simulink model "Ensamblaje2"  (R2018b)
settings: Solver=VariableStepAuto  StartTime=0.0  StopTime=30  RelTol=1e-6
model workspace: external: MATLAB File C:\matlabbb\EnsamblajePrueba_DataFile.m (data not in the file)
values from neighbouring files (symbols this model uses):
  m = [5.70044 3.22698 4.31272 2.07206 2.24665 1.60879]    [Modelo.m]    (also in robot_init.m; robotics_toolbox.m)
undefined symbols (not defined in the file or in its folder): smiData, X, Y, Z
libraries: sm_lib x40, nesl_utility x15, simulink x1
settings Model: Creator=aland  LastModifiedBy=aland

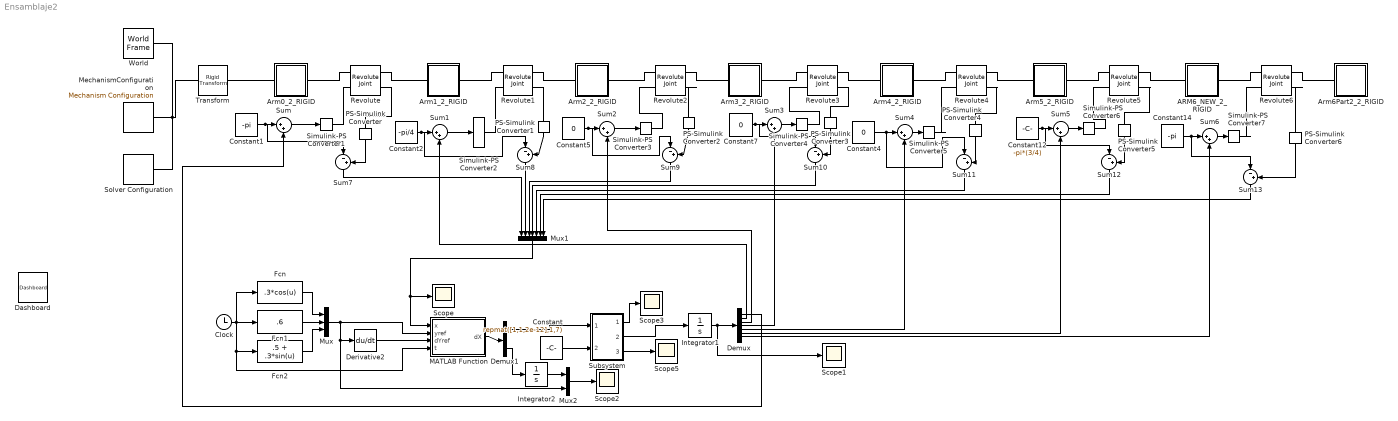
== system Ensamblaje2 ==
  ARM6_NEW_2_RIGID : Subsystem
  Arm0_2_RIGID : Subsystem
  Arm1_2_RIGID : Subsystem
  Arm2_2_RIGID : Subsystem
  Arm3_2_RIGID : Subsystem
  Arm4_2_RIGID : Subsystem
  Arm5_2_RIGID : Subsystem
  Arm6Part2_2_RIGID : Subsystem
  Clock : Clock
      settings: Decimation=10000
  Constant : Constant  Value=repmat([1,1,2e-12],1,7)
  Constant1 : Constant  Value=-pi
  Constant12 : Constant  Value=-pi*(3/4)
  Constant14 : Constant  Value=-pi
  Constant2 : Constant  Value=-pi/4
  Constant4 : Constant  Value=0
  Constant5 : Constant  Value=0
  Constant7 : Constant  Value=0
  Dashboard : simulink/Dashboard  SystemSampleTime=-1
      settings: SourceProductName=Simulink  SourceProductBaseCode=SL
  Demux : Demux  Outputs=7
  Demux1 : Demux  Outputs=[7 3]
  Derivative2 : Derivative
  Fcn : Fcn  Expr=.3*cos(u)
  Fcn1 : Fcn  Expr=.6
  Fcn2 : Fcn  Expr=.5 + .3*sin(u)
  Integrator1 : Integrator  InitialCondition=[0 0 0 0 0 0 0]  UpperSaturationLimit=4  LowerSaturationLimit=-4
  Integrator2 : Integrator  InitialCondition=[.148 0 1.2385]  UpperSaturationLimit=4  LowerSaturationLimit=-4
  MATLAB Function : MATLAB Function  TreatAsAtomicUnit=on
  MechanismConfiguration : sm_lib/Utilities/Mechanism Configuration  UniformGravity=Constant  GravityVector=[0 -9.80665 0]  GravityUnits=m/s^2  LinearizationDelta=0.001
  Mux : Mux  Inputs=3
  Mux1 : Mux  Inputs=7
  Mux2 : Mux  Inputs=2
  PS-Simulink Converter{,1..6} (7 alike) : nesl_utility/PS-Simulink Converter  PhysicalDomain=network_engine_domain  SubClassName=ps_output  LeftPortType=input  RightPortType=output  PseudoPeriodic=off  Frequencies=[]  Unit=1  AffineConversion=off
  Revolute{,1..4} (5 alike) : sm_lib/Joints/Revolute Joint  SenseConstraintForce=off  SenseConstraintForceX=off  SenseConstraintForceY=off  SenseConstraintForceZ=off  SenseConstraintTorque=off  SenseConstraintTorqueX=off  SenseConstraintTorqueY=off  SenseConstraintTorqueZ=off  SenseTotalForce=off  SenseTotalForceX=off  SenseTotalForceY=off  SenseTotalForceZ=off  SenseTotalTorque=off  SenseTotalTorqueX=off  SenseTotalTorqueY=off  SenseTotalTorqueZ=off  CompositeWrenchDir=FollowerOnBase  CompositeWrenchFrame=BaseFrame  EquilibriumPosition=0  EquilibriumPositionUnits=rad  SpringStiffness=0  SpringStiffnessUnits=N*m/rad  DampingCoefficient=0  DampingCoefficientUnits=N*m/(rad/s)  TorqueActuationMode=ComputedTorque  MotionActuationMode=InputMotion  SensePosition=on  SenseVelocity=off  SenseAcceleration=off  SenseTorqueForce=off  PositionTargetSpecify=off  PositionTargetPriority=Low  PositionTargetValue=0  PositionTargetValueUnits=deg  VelocityTargetSpecify=off  VelocityTargetPriority=High  VelocityTargetValue=0  VelocityTargetValueUnits=deg/s
  Revolute5 : sm_lib/Joints/Revolute Joint  SenseConstraintForce=off  SenseConstraintForceX=off  SenseConstraintForceY=off  SenseConstraintForceZ=off  SenseConstraintTorque=off  SenseConstraintTorqueX=off  SenseConstraintTorqueY=off  SenseConstraintTorqueZ=off  SenseTotalForce=off  SenseTotalForceX=off  SenseTotalForceY=off  SenseTotalForceZ=off  SenseTotalTorque=off  SenseTotalTorqueX=off  SenseTotalTorqueY=off  SenseTotalTorqueZ=off  CompositeWrenchDir=FollowerOnBase  CompositeWrenchFrame=BaseFrame  EquilibriumPosition=0  EquilibriumPositionUnits=rad  SpringStiffness=0  SpringStiffnessUnits=N*m/rad  DampingCoefficient=0  DampingCoefficientUnits=N*m/(rad/s)  TorqueActuationMode=ComputedTorque  MotionActuationMode=InputMotion  SensePosition=on  SenseVelocity=off  SenseAcceleration=off  SenseTorqueForce=off  PositionTargetSpecify=off  PositionTargetPriority=Low  PositionTargetValue=smiData.RevoluteJoint(6).Rz.Pos  PositionTargetValueUnits=deg  VelocityTargetSpecify=off  VelocityTargetPriority=High  VelocityTargetValue=0  VelocityTargetValueUnits=deg/s
  Revolute6 : sm_lib/Joints/Revolute Joint  SenseConstraintForce=off  SenseConstraintForceX=off  SenseConstraintForceY=off  SenseConstraintForceZ=off  SenseConstraintTorque=off  SenseConstraintTorqueX=off  SenseConstraintTorqueY=off  SenseConstraintTorqueZ=off  SenseTotalForce=off  SenseTotalForceX=off  SenseTotalForceY=off  SenseTotalForceZ=off  SenseTotalTorque=off  SenseTotalTorqueX=off  SenseTotalTorqueY=off  SenseTotalTorqueZ=off  CompositeWrenchDir=FollowerOnBase  CompositeWrenchFrame=BaseFrame  EquilibriumPosition=0  EquilibriumPositionUnits=rad  SpringStiffness=0  SpringStiffnessUnits=N*m/rad  DampingCoefficient=0  DampingCoefficientUnits=N*m/(rad/s)  TorqueActuationMode=ComputedTorque  MotionActuationMode=InputMotion  SensePosition=on  SenseVelocity=off  SenseAcceleration=off  SenseTorqueForce=off  PositionTargetSpecify=off  PositionTargetPriority=Low  PositionTargetValue=smiData.RevoluteJoint(7).Rz.Pos  PositionTargetValueUnits=deg  VelocityTargetSpecify=off  VelocityTargetPriority=High  VelocityTargetValue=0  VelocityTargetValueUnits=deg/s
  Scope{,1..3,5} (5 alike) : Scope
  Simulink-PS Converter{1..7} (7 alike) : nesl_utility/Simulink-PS Converter  PhysicalDomain=network_engine_domain  SubClassName=ps_input  LeftPortType=input  RightPortType=output  PseudoPeriodic=off  Frequencies=[]  NoiseDistribution=none  NoiseParameters=[]  Unit=1  AffineConversion=off  FilteringAndDerivatives=filter  SimscapeFilterOrder=2  InputFilterTimeConstant=0.0001  UdotUserProvided=0
  Solver Configuration : nesl_utility/Solver Configuration  PhysicalDomain=network_engine_domain  SubClassName=solver  LeftPortType=input  RightPortType=generic  Tones=[]  Harmonics=[]  SimulateNoise=off  Profile=off  UseLocalSampling=off  EnableSwitchedLinearOptims=on  FrequencyDomain=off  UseCCode=off  RelTol=0.001  AbsTol=1e-06  MinStep=1e-09  ToWorkspace=off  RevertToSquareIcSolve=off  NumHomotopyIterations=100  PhasorMode=off  PhasorModeNumHarmonics=1  DoDC=off  ResidualTolerance=1e-09  UseLocalSolver=off  LocalSolverChoice=NE_BACKWARD_EULER_ADVANCER  LocalSolverSampleTime=0.001  DoFixedCost=off  MaxNonlinIter=3  MaxModeIter=2  LinearAlgebra=auto  EquationFormulation=NE_TIME_EF  DelaysMemoryBudget=1024  AutomaticFiltering=on  FilteringTimeConstant=0.001  PartitionStorageMethod=AS_NEEDED  PartitionMemoryBudget=1024
  Subsystem : Subsystem
  Sum{,1..6} (7 alike) : Sum  Inputs=|++
  Sum{7..13} (7 alike) : Sum  Inputs=|-+
  Transform : sm_lib/Frames and Transforms/Rigid Transform  TranslationMethod=Cartesian  TranslationStandardOffset=0  TranslationLengthUnit=cm  TranslationStandardAxis=+Z  TranslationCartesianOffset=smiData.RigidTransform(15).translation  TranslationROffset=0  TranslationROffsetUnits=m  TranslationZOffset=0  TranslationZOffsetUnits=m  TranslationThetaOffset=0  TranslationThetaOffsetUnits=deg  RotationMethod=AlignedAxes  RotationAngleUnits=rad  RotationStandardAxis=+Z  RotationAngle=smiData.RigidTransform(15).angle  RotationArbitraryAxis=[180 90 90]  FollAlignAxisA=+Z  BaseAlignAxisA=+Y  FollAlignAxisB=+Y  BaseAlignAxisB=+Z  RotationSequenceAxes=FollowerAxes  RotationSequence=XYX  RotationSequenceAngles=[0 0 0]  RotationSequenceAnglesUnits=deg  RotationMatrix=[1 0 0; 0 1 0; 0 0 1]
  World : sm_lib/Frames and Transforms/World Frame
  wires:
  Constant1/1 -> Sum7/1, Sum/1
  Sum/1 -> Simulink-PS Converter1/1
  Sum1/1 -> Simulink-PS Converter2/1
  Constant2/1 -> Sum8/1, Sum1/1
  Constant5/1 -> Sum9/1, Sum2/1
  Sum2/1 -> Simulink-PS Converter3/1
  Sum3/1 -> Simulink-PS Converter4/1
  Constant7/1 -> Sum10/1, Sum3/1
  Constant12/1 -> Sum12/1, Sum5/1
  Sum5/1 -> Simulink-PS Converter6/1
  Constant14/1 -> Sum13/1, Sum6/1
  Sum6/1 -> Simulink-PS Converter7/1
  Mux1/1 -> Scope/1, MATLAB Function/1(x)
  Constant4/1 -> Sum11/1, Sum4/1
  Sum4/1 -> Simulink-PS Converter5/1
  Demux/1 -> Sum/2
  Demux/2 -> Sum1/2
  Demux/3 -> Sum2/2
  Demux/4 -> Sum3/2
  Demux/5 -> Sum4/2
  Demux/6 -> Sum5/2
  Integrator1/1 -> Scope1/1, Demux/1
  PS-Simulink Converter/1 -> Sum7/2
  Sum7/1 -> Mux1/1
  PS-Simulink Converter1/1 -> Sum8/2
  PS-Simulink Converter2/1 -> Sum9/2
  Sum8/1 -> Mux1/2
  Sum9/1 -> Mux1/3
  PS-Simulink Converter3/1 -> Sum10/2
  Sum10/1 -> Mux1/4
  PS-Simulink Converter4/1 -> Sum11/2
  Sum11/1 -> Mux1/5
  PS-Simulink Converter5/1 -> Sum12/2
  Sum12/1 -> Mux1/6
  PS-Simulink Converter6/1 -> Sum13/2
  Sum13/1 -> Mux1/7
  Clock/1 -> Fcn2/1, MATLAB Function/4(t), Fcn1/1, Fcn/1
  Mux/1 -> Mux2/2, Derivative2/1, MATLAB Function/2(yref)
  Derivative2/1 -> MATLAB Function/3(dYref)
  Fcn/1 -> Mux/1
  Fcn1/1 -> Mux/2
  Fcn2/1 -> Mux/3
  MATLAB Function/1(dX) -> Demux1/1
  Demux1/1 -> Subsystem/1(In1)
  Subsystem/1(Out1) -> Scope3/1
  Subsystem/2(Out2) -> Integrator1/1
  Constant/1 -> Subsystem/2(In2)
  Subsystem/3(Out3) -> Scope5/1
  Demux/7 -> Sum6/2
  Mux2/1 -> Scope2/1
  Demux1/2 -> Integrator2/1
  Integrator2/1 -> Mux2/1
  connections:
  Transform/LConn1 -- MechanismConfiguration/RConn1 -- Solver Configuration/RConn1 -- World/RConn1
  Arm0_2_RIGID/RConn1 -- Revolute/LConn1
  Arm5_2_RIGID/LConn1 -- Revolute4/RConn1
  Arm5_2_RIGID/RConn1 -- Revolute5/LConn1
  ARM6_NEW_2_RIGID/LConn1 -- Revolute5/RConn1
  ARM6_NEW_2_RIGID/RConn1 -- Revolute6/LConn1
  Arm6Part2_2_RIGID/LConn1 -- Revolute6/RConn1
  Arm0_2_RIGID/LConn1 -- Transform/RConn1
  Arm1_2_RIGID/LConn1 -- Revolute/RConn1
  Arm1_2_RIGID/RConn1 -- Revolute1/LConn1
  Arm2_2_RIGID/LConn1 -- Revolute1/RConn1
  Arm2_2_RIGID/RConn1 -- Revolute2/LConn1
  Arm3_2_RIGID/LConn1 -- Revolute2/RConn1
  Arm3_2_RIGID/RConn1 -- Revolute3/LConn1
  Arm4_2_RIGID/LConn1 -- Revolute3/RConn1
  Arm4_2_RIGID/RConn1 -- Revolute4/LConn1
  Simulink-PS Converter1/RConn1 -- Revolute/LConn2
  Simulink-PS Converter2/RConn1 -- Revolute1/LConn2
  Simulink-PS Converter3/RConn1 -- Revolute2/LConn2
  Simulink-PS Converter4/RConn1 -- Revolute3/LConn2
  Simulink-PS Converter6/RConn1 -- Revolute5/LConn2
  Simulink-PS Converter5/RConn1 -- Revolute4/LConn2
  Simulink-PS Converter7/RConn1 -- Revolute6/LConn2
  Revolute/RConn2 -- PS-Simulink Converter/LConn1
  Revolute1/RConn2 -- PS-Simulink Converter1/LConn1
  Revolute2/RConn2 -- PS-Simulink Converter2/LConn1
  Revolute3/RConn2 -- PS-Simulink Converter3/LConn1
  Revolute4/RConn2 -- PS-Simulink Converter4/LConn1
  Revolute5/RConn2 -- PS-Simulink Converter5/LConn1
  Revolute6/RConn2 -- PS-Simulink Converter6/LConn1

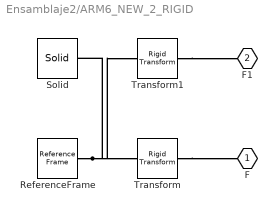
== system Ensamblaje2/ARM6_NEW_2_RIGID ==
  ReferenceFrame : sm_lib/Frames and Transforms/Reference Frame
  Solid : sm_lib/Body Elements/Solid  InertiaType=Custom  Mass=smiData.Solid(1).mass  MassUnits=kg  CenterOfMass=smiData.Solid(1).CoM  CenterOfMassUnits=cm  MomentsOfInertia=smiData.Solid(1).MoI  MomentsOfInertiaUnits=kg*cm^2  ProductsOfInertia=smiData.Solid(1).PoI  ProductsOfInertiaUnits=kg*cm^2  BasedOnType=Density  Density=1000  DensityUnits=kg/m^3  DoExposeReferenceFrame=on  SerializedFrames=<Frames/>  GraphicType=FromGeometry  MarkerShape=Sphere  MarkerSize=10  GraphicVisPropType=SimpleVisualProperties  GraphicDiffuseColor=smiData.Solid(1).color  GraphicSpecularColor=[0.5 0.5 0.5 1.0]  GraphicAmbientColor=[0.15 0.15 0.15 1.0]  GraphicEmissiveColor=[0.0 0.0 0.0 1.0]  GraphicShininess=75  GraphicOpacity=smiData.Solid(1).opacity  GeometryShape=FromFile  RectangleSize=[1 1]  RectangleSizeUnits=m  BrickDimensions=[1 1 1]  BrickDimensionUnits=m  CylinderRadius=1  CylinderRadiusUnits=m  CylinderLength=1  CylinderLengthUnits=m  SphereRadius=1  SphereRadiusUnits=m  EllipsoidRadii=[1 1 1]  EllipsoidRadiiUnits=m  ExtrusionCrossSection=[1 1; -1 1; -1 -1; 1 -1]  ExtrusionCrossSectionUnits=m  ExtrusionLength=1  ExtrusionLengthUnits=m  PolygonNumSides=3  PolygonOuterRadius=1  PolygonOuterRadiusUnits=m  ExtGeomFileType=STEP  ExtGeomFileName=ARM6_NEW_Default_sldprt.STEP  ExtGeomFileUnits=m  RevolutionCrossSection=[1 1; 1 -1; 2 -1; 2 1]  RevolutionCrossSectionUnits=m  RevolutionExtent=Full  RevolutionAngle=180  RevolutionAngleUnits=deg
  Transform : sm_lib/Frames and Transforms/Rigid Transform  TranslationMethod=Cartesian  TranslationStandardOffset=0  TranslationLengthUnit=cm  TranslationStandardAxis=+Z  TranslationCartesianOffset=smiData.RigidTransform(12).translation  TranslationROffset=0  TranslationROffsetUnits=m  TranslationZOffset=0  TranslationZOffsetUnits=m  TranslationThetaOffset=0  TranslationThetaOffsetUnits=deg  RotationMethod=ArbitraryAxis  RotationAngleUnits=rad  RotationStandardAxis=+Z  RotationAngle=smiData.RigidTransform(12).angle  RotationArbitraryAxis=smiData.RigidTransform(12).axis  FollAlignAxisA=+X  BaseAlignAxisA=+Y  FollAlignAxisB=+Y  BaseAlignAxisB=+Z  RotationSequenceAxes=FollowerAxes  RotationSequence=XYX  RotationSequenceAngles=[0 0 0]  RotationSequenceAnglesUnits=deg  RotationMatrix=[1 0 0; 0 1 0; 0 0 1]
  Transform1 : sm_lib/Frames and Transforms/Rigid Transform  TranslationMethod=Cartesian  TranslationStandardOffset=0  TranslationLengthUnit=cm  TranslationStandardAxis=+Z  TranslationCartesianOffset=smiData.RigidTransform(13).translation  TranslationROffset=0  TranslationROffsetUnits=m  TranslationZOffset=0  TranslationZOffsetUnits=m  TranslationThetaOffset=0  TranslationThetaOffsetUnits=deg  RotationMethod=ArbitraryAxis  RotationAngleUnits=rad  RotationStandardAxis=+Z  RotationAngle=smiData.RigidTransform(13).angle  RotationArbitraryAxis=smiData.RigidTransform(13).axis  FollAlignAxisA=+X  BaseAlignAxisA=+Y  FollAlignAxisB=+Y  BaseAlignAxisB=+Z  RotationSequenceAxes=FollowerAxes  RotationSequence=XYX  RotationSequenceAngles=[0 0 0]  RotationSequenceAnglesUnits=deg  RotationMatrix=[1 0 0; 0 1 0; 0 0 1]
  F : PMIOPort  Side=Left
  F1 : PMIOPort  Port=2  Side=Right
  connections:
  Solid/RConn1 -- ReferenceFrame/RConn1 -- Transform/LConn1 -- Transform1/LConn1
  Transform/RConn1 -- F/RConn1
  Transform1/RConn1 -- F1/RConn1

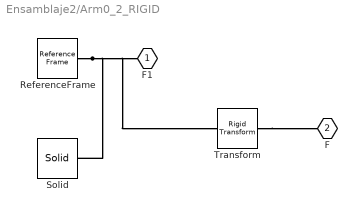
== system Ensamblaje2/Arm0_2_RIGID ==
  ReferenceFrame : sm_lib/Frames and Transforms/Reference Frame
  Solid : sm_lib/Body Elements/Solid  InertiaType=Custom  Mass=smiData.Solid(8).mass  MassUnits=kg  CenterOfMass=smiData.Solid(8).CoM  CenterOfMassUnits=in  MomentsOfInertia=smiData.Solid(8).MoI  MomentsOfInertiaUnits=kg*in^2  ProductsOfInertia=smiData.Solid(8).PoI  ProductsOfInertiaUnits=kg*in^2  BasedOnType=Density  Density=1000  DensityUnits=kg/m^3  DoExposeReferenceFrame=on  SerializedFrames=<Frames/>  GraphicType=FromGeometry  MarkerShape=Sphere  MarkerSize=10  GraphicVisPropType=SimpleVisualProperties  GraphicDiffuseColor=smiData.Solid(8).color  GraphicSpecularColor=[0.5 0.5 0.5 1.0]  GraphicAmbientColor=[0.15 0.15 0.15 1.0]  GraphicEmissiveColor=[0.0 0.0 0.0 1.0]  GraphicShininess=75  GraphicOpacity=smiData.Solid(8).opacity  GeometryShape=FromFile  RectangleSize=[1 1]  RectangleSizeUnits=m  BrickDimensions=[1 1 1]  BrickDimensionUnits=m  CylinderRadius=1  CylinderRadiusUnits=m  CylinderLength=1  CylinderLengthUnits=m  SphereRadius=1  SphereRadiusUnits=m  EllipsoidRadii=[1 1 1]  EllipsoidRadiiUnits=m  ExtrusionCrossSection=[1 1; -1 1; -1 -1; 1 -1]  ExtrusionCrossSectionUnits=m  ExtrusionLength=1  ExtrusionLengthUnits=m  PolygonNumSides=3  PolygonOuterRadius=1  PolygonOuterRadiusUnits=m  ExtGeomFileType=STEP  ExtGeomFileName=Arm0_Default_sldprt.STEP  ExtGeomFileUnits=m  RevolutionCrossSection=[1 1; 1 -1; 2 -1; 2 1]  RevolutionCrossSectionUnits=m  RevolutionExtent=Full  RevolutionAngle=180  RevolutionAngleUnits=deg
  Transform : sm_lib/Frames and Transforms/Rigid Transform  TranslationMethod=Cartesian  TranslationStandardOffset=0  TranslationLengthUnit=cm  TranslationStandardAxis=+Z  TranslationCartesianOffset=smiData.RigidTransform(1).translation  TranslationROffset=0  TranslationROffsetUnits=m  TranslationZOffset=0  TranslationZOffsetUnits=m  TranslationThetaOffset=0  TranslationThetaOffsetUnits=deg  RotationMethod=ArbitraryAxis  RotationAngleUnits=rad  RotationStandardAxis=+Z  RotationAngle=smiData.RigidTransform(1).angle  RotationArbitraryAxis=smiData.RigidTransform(1).axis  FollAlignAxisA=+X  BaseAlignAxisA=+Y  FollAlignAxisB=+Y  BaseAlignAxisB=+Z  RotationSequenceAxes=FollowerAxes  RotationSequence=XYX  RotationSequenceAngles=[0 0 0]  RotationSequenceAnglesUnits=deg  RotationMatrix=[1 0 0; 0 1 0; 0 0 1]
  F1 : PMIOPort  Side=Left
  F : PMIOPort  Port=2  Side=Right
  connections:
  Solid/RConn1 -- ReferenceFrame/RConn1 -- Transform/LConn1 -- F1/RConn1
  Transform/RConn1 -- F/RConn1

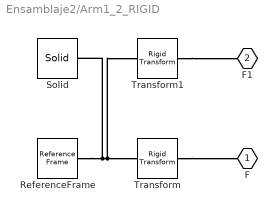
== system Ensamblaje2/Arm1_2_RIGID ==
  ReferenceFrame : sm_lib/Frames and Transforms/Reference Frame
  Solid : sm_lib/Body Elements/Solid  InertiaType=Custom  Mass=smiData.Solid(3).mass  MassUnits=kg  CenterOfMass=smiData.Solid(3).CoM  CenterOfMassUnits=in  MomentsOfInertia=smiData.Solid(3).MoI  MomentsOfInertiaUnits=kg*in^2  ProductsOfInertia=smiData.Solid(3).PoI  ProductsOfInertiaUnits=kg*in^2  BasedOnType=Density  Density=1000  DensityUnits=kg/m^3  DoExposeReferenceFrame=on  SerializedFrames=<Frames/>  GraphicType=FromGeometry  MarkerShape=Sphere  MarkerSize=10  GraphicVisPropType=SimpleVisualProperties  GraphicDiffuseColor=smiData.Solid(3).color  GraphicSpecularColor=[0.5 0.5 0.5 1.0]  GraphicAmbientColor=[0.15 0.15 0.15 1.0]  GraphicEmissiveColor=[0.0 0.0 0.0 1.0]  GraphicShininess=75  GraphicOpacity=smiData.Solid(3).opacity  GeometryShape=FromFile  RectangleSize=[1 1]  RectangleSizeUnits=m  BrickDimensions=[1 1 1]  BrickDimensionUnits=m  CylinderRadius=1  CylinderRadiusUnits=m  CylinderLength=1  CylinderLengthUnits=m  SphereRadius=1  SphereRadiusUnits=m  EllipsoidRadii=[1 1 1]  EllipsoidRadiiUnits=m  ExtrusionCrossSection=[1 1; -1 1; -1 -1; 1 -1]  ExtrusionCrossSectionUnits=m  ExtrusionLength=1  ExtrusionLengthUnits=m  PolygonNumSides=3  PolygonOuterRadius=1  PolygonOuterRadiusUnits=m  ExtGeomFileType=STEP  ExtGeomFileName=Arm1_Default_sldprt.STEP  ExtGeomFileUnits=m  RevolutionCrossSection=[1 1; 1 -1; 2 -1; 2 1]  RevolutionCrossSectionUnits=m  RevolutionExtent=Full  RevolutionAngle=180  RevolutionAngleUnits=deg
  Transform : sm_lib/Frames and Transforms/Rigid Transform  TranslationMethod=Cartesian  TranslationStandardOffset=0  TranslationLengthUnit=cm  TranslationStandardAxis=+Z  TranslationCartesianOffset=smiData.RigidTransform(2).translation  TranslationROffset=0  TranslationROffsetUnits=m  TranslationZOffset=0  TranslationZOffsetUnits=m  TranslationThetaOffset=0  TranslationThetaOffsetUnits=deg  RotationMethod=ArbitraryAxis  RotationAngleUnits=rad  RotationStandardAxis=+Z  RotationAngle=smiData.RigidTransform(2).angle  RotationArbitraryAxis=smiData.RigidTransform(2).axis  FollAlignAxisA=+X  BaseAlignAxisA=+Y  FollAlignAxisB=+Y  BaseAlignAxisB=+Z  RotationSequenceAxes=FollowerAxes  RotationSequence=XYX  RotationSequenceAngles=[0 0 0]  RotationSequenceAnglesUnits=deg  RotationMatrix=[1 0 0; 0 1 0; 0 0 1]
  Transform1 : sm_lib/Frames and Transforms/Rigid Transform  TranslationMethod=Cartesian  TranslationStandardOffset=0  TranslationLengthUnit=cm  TranslationStandardAxis=+Z  TranslationCartesianOffset=smiData.RigidTransform(3).translation  TranslationROffset=0  TranslationROffsetUnits=m  TranslationZOffset=0  TranslationZOffsetUnits=m  TranslationThetaOffset=0  TranslationThetaOffsetUnits=deg  RotationMethod=ArbitraryAxis  RotationAngleUnits=rad  RotationStandardAxis=+Z  RotationAngle=smiData.RigidTransform(3).angle  RotationArbitraryAxis=smiData.RigidTransform(3).axis  FollAlignAxisA=+X  BaseAlignAxisA=+Y  FollAlignAxisB=+Y  BaseAlignAxisB=+Z  RotationSequenceAxes=FollowerAxes  RotationSequence=XYX  RotationSequenceAngles=[0 0 0]  RotationSequenceAnglesUnits=deg  RotationMatrix=[1 0 0; 0 1 0; 0 0 1]
  F : PMIOPort  Side=Left
  F1 : PMIOPort  Port=2  Side=Right
  connections:
  Solid/RConn1 -- ReferenceFrame/RConn1 -- Transform/LConn1 -- Transform1/LConn1
  Transform/RConn1 -- F/RConn1
  Transform1/RConn1 -- F1/RConn1

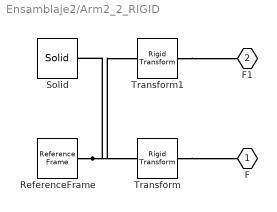
== system Ensamblaje2/Arm2_2_RIGID ==
  ReferenceFrame : sm_lib/Frames and Transforms/Reference Frame
  Solid : sm_lib/Body Elements/Solid  InertiaType=Custom  Mass=smiData.Solid(7).mass  MassUnits=kg  CenterOfMass=smiData.Solid(7).CoM  CenterOfMassUnits=in  MomentsOfInertia=smiData.Solid(7).MoI  MomentsOfInertiaUnits=kg*in^2  ProductsOfInertia=smiData.Solid(7).PoI  ProductsOfInertiaUnits=kg*in^2  BasedOnType=Density  Density=1000  DensityUnits=kg/m^3  DoExposeReferenceFrame=on  SerializedFrames=<Frames/>  GraphicType=FromGeometry  MarkerShape=Sphere  MarkerSize=10  GraphicVisPropType=SimpleVisualProperties  GraphicDiffuseColor=smiData.Solid(7).color  GraphicSpecularColor=[0.5 0.5 0.5 1.0]  GraphicAmbientColor=[0.15 0.15 0.15 1.0]  GraphicEmissiveColor=[0.0 0.0 0.0 1.0]  GraphicShininess=75  GraphicOpacity=smiData.Solid(7).opacity  GeometryShape=FromFile  RectangleSize=[1 1]  RectangleSizeUnits=m  BrickDimensions=[1 1 1]  BrickDimensionUnits=m  CylinderRadius=1  CylinderRadiusUnits=m  CylinderLength=1  CylinderLengthUnits=m  SphereRadius=1  SphereRadiusUnits=m  EllipsoidRadii=[1 1 1]  EllipsoidRadiiUnits=m  ExtrusionCrossSection=[1 1; -1 1; -1 -1; 1 -1]  ExtrusionCrossSectionUnits=m  ExtrusionLength=1  ExtrusionLengthUnits=m  PolygonNumSides=3  PolygonOuterRadius=1  PolygonOuterRadiusUnits=m  ExtGeomFileType=STEP  ExtGeomFileName=Arm2_Default_sldprt.STEP  ExtGeomFileUnits=m  RevolutionCrossSection=[1 1; 1 -1; 2 -1; 2 1]  RevolutionCrossSectionUnits=m  RevolutionExtent=Full  RevolutionAngle=180  RevolutionAngleUnits=deg
  Transform : sm_lib/Frames and Transforms/Rigid Transform  TranslationMethod=Cartesian  TranslationStandardOffset=0  TranslationLengthUnit=cm  TranslationStandardAxis=+Z  TranslationCartesianOffset=smiData.RigidTransform(4).translation  TranslationROffset=0  TranslationROffsetUnits=m  TranslationZOffset=0  TranslationZOffsetUnits=m  TranslationThetaOffset=0  TranslationThetaOffsetUnits=deg  RotationMethod=ArbitraryAxis  RotationAngleUnits=rad  RotationStandardAxis=+Z  RotationAngle=smiData.RigidTransform(4).angle  RotationArbitraryAxis=smiData.RigidTransform(4).axis  FollAlignAxisA=+X  BaseAlignAxisA=+Y  FollAlignAxisB=+Y  BaseAlignAxisB=+Z  RotationSequenceAxes=FollowerAxes  RotationSequence=XYX  RotationSequenceAngles=[0 0 0]  RotationSequenceAnglesUnits=deg  RotationMatrix=[1 0 0; 0 1 0; 0 0 1]
  Transform1 : sm_lib/Frames and Transforms/Rigid Transform  TranslationMethod=Cartesian  TranslationStandardOffset=0  TranslationLengthUnit=cm  TranslationStandardAxis=+Z  TranslationCartesianOffset=smiData.RigidTransform(5).translation  TranslationROffset=0  TranslationROffsetUnits=m  TranslationZOffset=0  TranslationZOffsetUnits=m  TranslationThetaOffset=0  TranslationThetaOffsetUnits=deg  RotationMethod=ArbitraryAxis  RotationAngleUnits=rad  RotationStandardAxis=+Z  RotationAngle=smiData.RigidTransform(5).angle  RotationArbitraryAxis=smiData.RigidTransform(5).axis  FollAlignAxisA=+X  BaseAlignAxisA=+Y  FollAlignAxisB=+Y  BaseAlignAxisB=+Z  RotationSequenceAxes=FollowerAxes  RotationSequence=XYX  RotationSequenceAngles=[0 0 0]  RotationSequenceAnglesUnits=deg  RotationMatrix=[1 0 0; 0 1 0; 0 0 1]
  F : PMIOPort  Side=Left
  F1 : PMIOPort  Port=2  Side=Right
  connections:
  Solid/RConn1 -- ReferenceFrame/RConn1 -- Transform/LConn1 -- Transform1/LConn1
  Transform/RConn1 -- F/RConn1
  Transform1/RConn1 -- F1/RConn1

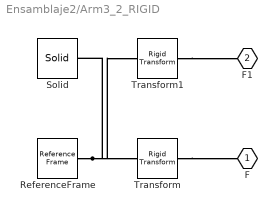
== system Ensamblaje2/Arm3_2_RIGID ==
  ReferenceFrame : sm_lib/Frames and Transforms/Reference Frame
  Solid : sm_lib/Body Elements/Solid  InertiaType=Custom  Mass=smiData.Solid(5).mass  MassUnits=kg  CenterOfMass=smiData.Solid(5).CoM  CenterOfMassUnits=in  MomentsOfInertia=smiData.Solid(5).MoI  MomentsOfInertiaUnits=kg*in^2  ProductsOfInertia=smiData.Solid(5).PoI  ProductsOfInertiaUnits=kg*in^2  BasedOnType=Density  Density=1000  DensityUnits=kg/m^3  DoExposeReferenceFrame=on  SerializedFrames=<Frames/>  GraphicType=FromGeometry  MarkerShape=Sphere  MarkerSize=10  GraphicVisPropType=SimpleVisualProperties  GraphicDiffuseColor=smiData.Solid(5).color  GraphicSpecularColor=[0.5 0.5 0.5 1.0]  GraphicAmbientColor=[0.15 0.15 0.15 1.0]  GraphicEmissiveColor=[0.0 0.0 0.0 1.0]  GraphicShininess=75  GraphicOpacity=smiData.Solid(5).opacity  GeometryShape=FromFile  RectangleSize=[1 1]  RectangleSizeUnits=m  BrickDimensions=[1 1 1]  BrickDimensionUnits=m  CylinderRadius=1  CylinderRadiusUnits=m  CylinderLength=1  CylinderLengthUnits=m  SphereRadius=1  SphereRadiusUnits=m  EllipsoidRadii=[1 1 1]  EllipsoidRadiiUnits=m  ExtrusionCrossSection=[1 1; -1 1; -1 -1; 1 -1]  ExtrusionCrossSectionUnits=m  ExtrusionLength=1  ExtrusionLengthUnits=m  PolygonNumSides=3  PolygonOuterRadius=1  PolygonOuterRadiusUnits=m  ExtGeomFileType=STEP  ExtGeomFileName=Arm3_Default_sldprt.STEP  ExtGeomFileUnits=m  RevolutionCrossSection=[1 1; 1 -1; 2 -1; 2 1]  RevolutionCrossSectionUnits=m  RevolutionExtent=Full  RevolutionAngle=180  RevolutionAngleUnits=deg
  Transform : sm_lib/Frames and Transforms/Rigid Transform  TranslationMethod=Cartesian  TranslationStandardOffset=0  TranslationLengthUnit=cm  TranslationStandardAxis=+Z  TranslationCartesianOffset=smiData.RigidTransform(6).translation  TranslationROffset=0  TranslationROffsetUnits=m  TranslationZOffset=0  TranslationZOffsetUnits=m  TranslationThetaOffset=0  TranslationThetaOffsetUnits=deg  RotationMethod=ArbitraryAxis  RotationAngleUnits=rad  RotationStandardAxis=+Z  RotationAngle=smiData.RigidTransform(6).angle  RotationArbitraryAxis=smiData.RigidTransform(6).axis  FollAlignAxisA=+X  BaseAlignAxisA=+Y  FollAlignAxisB=+Y  BaseAlignAxisB=+Z  RotationSequenceAxes=FollowerAxes  RotationSequence=XYX  RotationSequenceAngles=[0 0 0]  RotationSequenceAnglesUnits=deg  RotationMatrix=[1 0 0; 0 1 0; 0 0 1]
  Transform1 : sm_lib/Frames and Transforms/Rigid Transform  TranslationMethod=Cartesian  TranslationStandardOffset=0  TranslationLengthUnit=cm  TranslationStandardAxis=+Z  TranslationCartesianOffset=smiData.RigidTransform(7).translation  TranslationROffset=0  TranslationROffsetUnits=m  TranslationZOffset=0  TranslationZOffsetUnits=m  TranslationThetaOffset=0  TranslationThetaOffsetUnits=deg  RotationMethod=ArbitraryAxis  RotationAngleUnits=rad  RotationStandardAxis=+Z  RotationAngle=smiData.RigidTransform(7).angle  RotationArbitraryAxis=smiData.RigidTransform(7).axis  FollAlignAxisA=+X  BaseAlignAxisA=+Y  FollAlignAxisB=+Y  BaseAlignAxisB=+Z  RotationSequenceAxes=FollowerAxes  RotationSequence=XYX  RotationSequenceAngles=[0 0 0]  RotationSequenceAnglesUnits=deg  RotationMatrix=[1 0 0; 0 1 0; 0 0 1]
  F : PMIOPort  Side=Left
  F1 : PMIOPort  Port=2  Side=Right
  connections:
  Solid/RConn1 -- ReferenceFrame/RConn1 -- Transform/LConn1 -- Transform1/LConn1
  Transform/RConn1 -- F/RConn1
  Transform1/RConn1 -- F1/RConn1

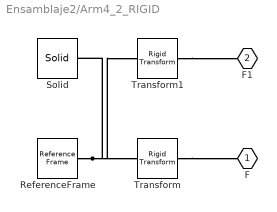
== system Ensamblaje2/Arm4_2_RIGID ==
  ReferenceFrame : sm_lib/Frames and Transforms/Reference Frame
  Solid : sm_lib/Body Elements/Solid  InertiaType=Custom  Mass=smiData.Solid(4).mass  MassUnits=kg  CenterOfMass=smiData.Solid(4).CoM  CenterOfMassUnits=in  MomentsOfInertia=smiData.Solid(4).MoI  MomentsOfInertiaUnits=kg*in^2  ProductsOfInertia=smiData.Solid(4).PoI  ProductsOfInertiaUnits=kg*in^2  BasedOnType=Density  Density=1000  DensityUnits=kg/m^3  DoExposeReferenceFrame=on  SerializedFrames=<Frames/>  GraphicType=FromGeometry  MarkerShape=Sphere  MarkerSize=10  GraphicVisPropType=SimpleVisualProperties  GraphicDiffuseColor=smiData.Solid(4).color  GraphicSpecularColor=[0.5 0.5 0.5 1.0]  GraphicAmbientColor=[0.15 0.15 0.15 1.0]  GraphicEmissiveColor=[0.0 0.0 0.0 1.0]  GraphicShininess=75  GraphicOpacity=smiData.Solid(4).opacity  GeometryShape=FromFile  RectangleSize=[1 1]  RectangleSizeUnits=m  BrickDimensions=[1 1 1]  BrickDimensionUnits=m  CylinderRadius=1  CylinderRadiusUnits=m  CylinderLength=1  CylinderLengthUnits=m  SphereRadius=1  SphereRadiusUnits=m  EllipsoidRadii=[1 1 1]  EllipsoidRadiiUnits=m  ExtrusionCrossSection=[1 1; -1 1; -1 -1; 1 -1]  ExtrusionCrossSectionUnits=m  ExtrusionLength=1  ExtrusionLengthUnits=m  PolygonNumSides=3  PolygonOuterRadius=1  PolygonOuterRadiusUnits=m  ExtGeomFileType=STEP  ExtGeomFileName=Arm4_Default_sldprt.STEP  ExtGeomFileUnits=m  RevolutionCrossSection=[1 1; 1 -1; 2 -1; 2 1]  RevolutionCrossSectionUnits=m  RevolutionExtent=Full  RevolutionAngle=180  RevolutionAngleUnits=deg
  Transform : sm_lib/Frames and Transforms/Rigid Transform  TranslationMethod=Cartesian  TranslationStandardOffset=0  TranslationLengthUnit=cm  TranslationStandardAxis=+Z  TranslationCartesianOffset=smiData.RigidTransform(8).translation  TranslationROffset=0  TranslationROffsetUnits=m  TranslationZOffset=0  TranslationZOffsetUnits=m  TranslationThetaOffset=0  TranslationThetaOffsetUnits=deg  RotationMethod=ArbitraryAxis  RotationAngleUnits=rad  RotationStandardAxis=+Z  RotationAngle=smiData.RigidTransform(8).angle  RotationArbitraryAxis=smiData.RigidTransform(8).axis  FollAlignAxisA=+X  BaseAlignAxisA=+Y  FollAlignAxisB=+Y  BaseAlignAxisB=+Z  RotationSequenceAxes=FollowerAxes  RotationSequence=XYX  RotationSequenceAngles=[0 0 0]  RotationSequenceAnglesUnits=deg  RotationMatrix=[1 0 0; 0 1 0; 0 0 1]
  Transform1 : sm_lib/Frames and Transforms/Rigid Transform  TranslationMethod=Cartesian  TranslationStandardOffset=0  TranslationLengthUnit=cm  TranslationStandardAxis=+Z  TranslationCartesianOffset=smiData.RigidTransform(9).translation  TranslationROffset=0  TranslationROffsetUnits=m  TranslationZOffset=0  TranslationZOffsetUnits=m  TranslationThetaOffset=0  TranslationThetaOffsetUnits=deg  RotationMethod=ArbitraryAxis  RotationAngleUnits=rad  RotationStandardAxis=+Z  RotationAngle=smiData.RigidTransform(9).angle  RotationArbitraryAxis=smiData.RigidTransform(9).axis  FollAlignAxisA=+X  BaseAlignAxisA=+Y  FollAlignAxisB=+Y  BaseAlignAxisB=+Z  RotationSequenceAxes=FollowerAxes  RotationSequence=XYX  RotationSequenceAngles=[0 0 0]  RotationSequenceAnglesUnits=deg  RotationMatrix=[1 0 0; 0 1 0; 0 0 1]
  F : PMIOPort  Side=Left
  F1 : PMIOPort  Port=2  Side=Right
  connections:
  Solid/RConn1 -- ReferenceFrame/RConn1 -- Transform/LConn1 -- Transform1/LConn1
  Transform/RConn1 -- F/RConn1
  Transform1/RConn1 -- F1/RConn1

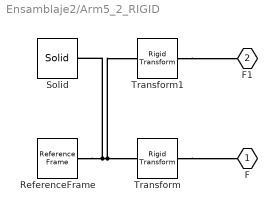
== system Ensamblaje2/Arm5_2_RIGID ==
  ReferenceFrame : sm_lib/Frames and Transforms/Reference Frame
  Solid : sm_lib/Body Elements/Solid  InertiaType=Custom  Mass=smiData.Solid(2).mass  MassUnits=kg  CenterOfMass=smiData.Solid(2).CoM  CenterOfMassUnits=in  MomentsOfInertia=smiData.Solid(2).MoI  MomentsOfInertiaUnits=kg*in^2  ProductsOfInertia=smiData.Solid(2).PoI  ProductsOfInertiaUnits=kg*in^2  BasedOnType=Density  Density=1000  DensityUnits=kg/m^3  DoExposeReferenceFrame=on  SerializedFrames=<Frames/>  GraphicType=FromGeometry  MarkerShape=Sphere  MarkerSize=10  GraphicVisPropType=SimpleVisualProperties  GraphicDiffuseColor=[0.4 0.4 0.4]  GraphicSpecularColor=[0.5 0.5 0.5 1.0]  GraphicAmbientColor=[0.15 0.15 0.15 1.0]  GraphicEmissiveColor=[0.0 0.0 0.0 1.0]  GraphicShininess=75  GraphicOpacity=1  GeometryShape=FromFile  RectangleSize=[1 1]  RectangleSizeUnits=m  BrickDimensions=[1 1 1]  BrickDimensionUnits=m  CylinderRadius=1  CylinderRadiusUnits=m  CylinderLength=1  CylinderLengthUnits=m  SphereRadius=1  SphereRadiusUnits=m  EllipsoidRadii=[1 1 1]  EllipsoidRadiiUnits=m  ExtrusionCrossSection=[1 1; -1 1; -1 -1; 1 -1]  ExtrusionCrossSectionUnits=m  ExtrusionLength=1  ExtrusionLengthUnits=m  PolygonNumSides=3  PolygonOuterRadius=1  PolygonOuterRadiusUnits=m  ExtGeomFileType=STEP  ExtGeomFileName=Arm5_Default_sldprt.STEP  ExtGeomFileUnits=m  RevolutionCrossSection=[1 1; 1 -1; 2 -1; 2 1]  RevolutionCrossSectionUnits=m  RevolutionExtent=Full  RevolutionAngle=180  RevolutionAngleUnits=deg
  Transform : sm_lib/Frames and Transforms/Rigid Transform  TranslationMethod=Cartesian  TranslationStandardOffset=0  TranslationLengthUnit=cm  TranslationStandardAxis=+Z  TranslationCartesianOffset=smiData.RigidTransform(10).translation  TranslationROffset=0  TranslationROffsetUnits=m  TranslationZOffset=0  TranslationZOffsetUnits=m  TranslationThetaOffset=0  TranslationThetaOffsetUnits=deg  RotationMethod=ArbitraryAxis  RotationAngleUnits=rad  RotationStandardAxis=+Z  RotationAngle=smiData.RigidTransform(10).angle  RotationArbitraryAxis=smiData.RigidTransform(10).axis  FollAlignAxisA=+X  BaseAlignAxisA=+Y  FollAlignAxisB=+Y  BaseAlignAxisB=+Z  RotationSequenceAxes=FollowerAxes  RotationSequence=XYX  RotationSequenceAngles=[0 0 0]  RotationSequenceAnglesUnits=deg  RotationMatrix=[1 0 0; 0 1 0; 0 0 1]
  Transform1 : sm_lib/Frames and Transforms/Rigid Transform  TranslationMethod=Cartesian  TranslationStandardOffset=0  TranslationLengthUnit=cm  TranslationStandardAxis=+Z  TranslationCartesianOffset=smiData.RigidTransform(11).translation  TranslationROffset=0  TranslationROffsetUnits=m  TranslationZOffset=0  TranslationZOffsetUnits=m  TranslationThetaOffset=0  TranslationThetaOffsetUnits=deg  RotationMethod=ArbitraryAxis  RotationAngleUnits=rad  RotationStandardAxis=+Z  RotationAngle=smiData.RigidTransform(11).angle  RotationArbitraryAxis=smiData.RigidTransform(11).axis  FollAlignAxisA=+X  BaseAlignAxisA=+Y  FollAlignAxisB=+Y  BaseAlignAxisB=+Z  RotationSequenceAxes=FollowerAxes  RotationSequence=XYX  RotationSequenceAngles=[0 0 0]  RotationSequenceAnglesUnits=deg  RotationMatrix=[1 0 0; 0 1 0; 0 0 1]
  F : PMIOPort  Side=Left
  F1 : PMIOPort  Port=2  Side=Right
  connections:
  Solid/RConn1 -- ReferenceFrame/RConn1 -- Transform/LConn1 -- Transform1/LConn1
  Transform/RConn1 -- F/RConn1
  Transform1/RConn1 -- F1/RConn1

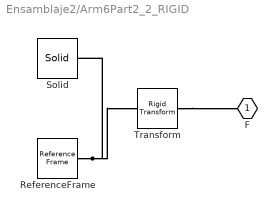
== system Ensamblaje2/Arm6Part2_2_RIGID ==
  ReferenceFrame : sm_lib/Frames and Transforms/Reference Frame
  Solid : sm_lib/Body Elements/Solid  InertiaType=Custom  Mass=smiData.Solid(6).mass  MassUnits=kg  CenterOfMass=smiData.Solid(6).CoM  CenterOfMassUnits=cm  MomentsOfInertia=smiData.Solid(6).MoI  MomentsOfInertiaUnits=kg*cm^2  ProductsOfInertia=smiData.Solid(6).PoI  ProductsOfInertiaUnits=kg*cm^2  BasedOnType=Density  Density=1000  DensityUnits=kg/m^3  DoExposeReferenceFrame=on  SerializedFrames=<Frames/>  GraphicType=FromGeometry  MarkerShape=Sphere  MarkerSize=10  GraphicVisPropType=SimpleVisualProperties  GraphicDiffuseColor=smiData.Solid(6).color  GraphicSpecularColor=[0.5 0.5 0.5 1.0]  GraphicAmbientColor=[0.15 0.15 0.15 1.0]  GraphicEmissiveColor=[0.0 0.0 0.0 1.0]  GraphicShininess=75  GraphicOpacity=smiData.Solid(6).opacity  GeometryShape=FromFile  RectangleSize=[1 1]  RectangleSizeUnits=m  BrickDimensions=[1 1 1]  BrickDimensionUnits=m  CylinderRadius=1  CylinderRadiusUnits=m  CylinderLength=1  CylinderLengthUnits=m  SphereRadius=1  SphereRadiusUnits=m  EllipsoidRadii=[1 1 1]  EllipsoidRadiiUnits=m  ExtrusionCrossSection=[1 1; -1 1; -1 -1; 1 -1]  ExtrusionCrossSectionUnits=m  ExtrusionLength=1  ExtrusionLengthUnits=m  PolygonNumSides=3  PolygonOuterRadius=1  PolygonOuterRadiusUnits=m  ExtGeomFileType=STEP  ExtGeomFileName=Arm6Part2_Default_sldprt.STEP  ExtGeomFileUnits=m  RevolutionCrossSection=[1 1; 1 -1; 2 -1; 2 1]  RevolutionCrossSectionUnits=m  RevolutionExtent=Full  RevolutionAngle=180  RevolutionAngleUnits=deg
  Transform : sm_lib/Frames and Transforms/Rigid Transform  TranslationMethod=Cartesian  TranslationStandardOffset=0  TranslationLengthUnit=cm  TranslationStandardAxis=+Z  TranslationCartesianOffset=smiData.RigidTransform(14).translation  TranslationROffset=0  TranslationROffsetUnits=m  TranslationZOffset=0  TranslationZOffsetUnits=m  TranslationThetaOffset=0  TranslationThetaOffsetUnits=deg  RotationMethod=ArbitraryAxis  RotationAngleUnits=rad  RotationStandardAxis=+Z  RotationAngle=smiData.RigidTransform(14).angle  RotationArbitraryAxis=smiData.RigidTransform(14).axis  FollAlignAxisA=+X  BaseAlignAxisA=+Y  FollAlignAxisB=+Y  BaseAlignAxisB=+Z  RotationSequenceAxes=FollowerAxes  RotationSequence=XYX  RotationSequenceAngles=[0 0 0]  RotationSequenceAnglesUnits=deg  RotationMatrix=[1 0 0; 0 1 0; 0 0 1]
  F : PMIOPort  Side=Left
  connections:
  Solid/RConn1 -- ReferenceFrame/RConn1 -- Transform/LConn1
  Transform/RConn1 -- F/RConn1

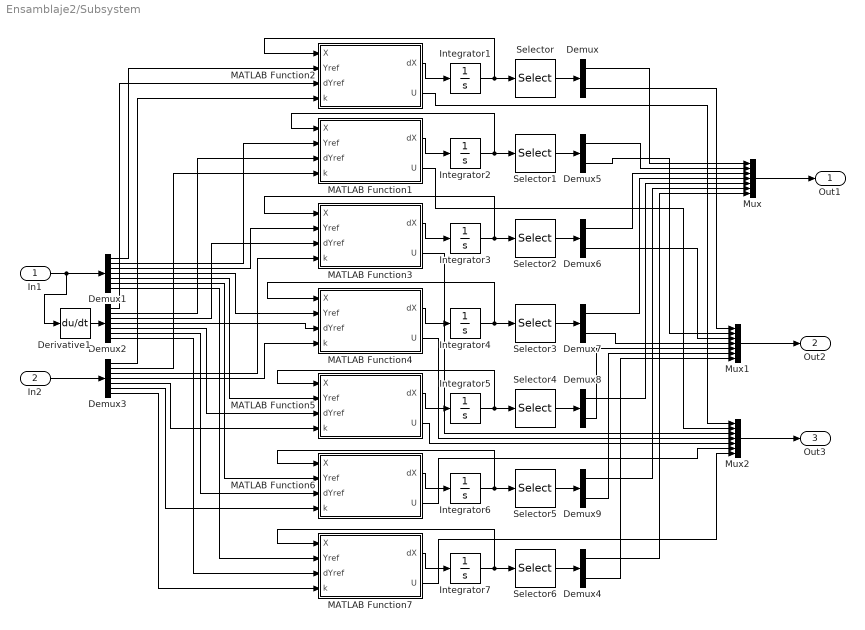
== system Ensamblaje2/Subsystem ==
  In1 : Inport
  In2 : Inport  Port=2
  Demux{,4..9} (7 alike) : Demux  Outputs=2
  Demux1 : Demux  Outputs=7
  Demux2 : Demux  Outputs=7
  Demux3 : Demux  Outputs=[3 3 3 3 3 3 3]
  Derivative1 : Derivative
  Integrator{1..7} (7 alike) : Integrator  InitialCondition=[0 0 0]
  MATLAB Function1 : MATLAB Function  TreatAsAtomicUnit=on
  MATLAB Function2 : MATLAB Function  TreatAsAtomicUnit=on
  MATLAB Function3 : MATLAB Function  TreatAsAtomicUnit=on
  MATLAB Function4 : MATLAB Function  TreatAsAtomicUnit=on
  MATLAB Function5 : MATLAB Function  TreatAsAtomicUnit=on
  MATLAB Function6 : MATLAB Function  TreatAsAtomicUnit=on
  MATLAB Function7 : MATLAB Function  TreatAsAtomicUnit=on
  Mux : Mux  Inputs=7
  Mux1 : Mux  Inputs=7
  Mux2 : Mux  Inputs=7
  Selector{,1..6} (7 alike) : Selector  InputPortWidth=3  IndexOptions=Index vector (dialog)  Indices=[2:3]  OutputSizes=1
  Out1 : Outport
  Out2 : Outport  Port=2
  Out3 : Outport  Port=3
  wires:
  In2/1 -> Demux3/1
  Demux4/2 -> Mux1/7
  Demux3/6 -> MATLAB Function6/4(k)
  Demux3/2 -> MATLAB Function1/4(k)
  Demux3/4 -> MATLAB Function4/4(k)
  Integrator4/1 -> Selector3/1, MATLAB Function4/1(X)
  Demux5/2 -> Mux1/2
  MATLAB Function3/1(dX) -> Integrator3/1
  MATLAB Function6/1(dX) -> Integrator6/1
  Demux5/1 -> Mux/2
  Integrator2/1 -> Selector1/1, MATLAB Function1/1(X)
  Integrator1/1 -> MATLAB Function2/1(X), Selector/1
  Demux2/7 -> MATLAB Function7/3(dYref)
  MATLAB Function4/1(dX) -> Integrator4/1
  Demux2/1 -> MATLAB Function2/3(dYref)
  Demux3/5 -> MATLAB Function5/4(k)
  Demux1/5 -> MATLAB Function5/2(Yref)
  Integrator6/1 -> Selector5/1, MATLAB Function6/1(X)
  Demux2/3 -> MATLAB Function3/3(dYref)
  Integrator3/1 -> Selector2/1, MATLAB Function3/1(X)
  Demux2/5 -> MATLAB Function5/3(dYref)
  Demux1/4 -> MATLAB Function4/2(Yref)
  MATLAB Function1/1(dX) -> Integrator2/1
  Demux1/6 -> MATLAB Function6/2(Yref)
  Demux7/1 -> Mux/4
  MATLAB Function5/1(dX) -> Integrator5/1
  Integrator5/1 -> Selector4/1, MATLAB Function5/1(X)
  Demux6/1 -> Mux/3
  MATLAB Function7/1(dX) -> Integrator7/1
  Demux1/7 -> MATLAB Function7/2(Yref)
  Demux3/7 -> MATLAB Function7/4(k)
  Demux9/2 -> Mux1/6
  Integrator7/1 -> Selector6/1, MATLAB Function7/1(X)
  Demux1/1 -> MATLAB Function2/2(Yref)
  Demux8/2 -> Mux1/5
  Demux6/2 -> Mux1/3
  Demux3/3 -> MATLAB Function3/4(k)
  Demux7/2 -> Mux1/4
  Demux2/6 -> MATLAB Function6/3(dYref)
  Demux/2 -> Mux1/1
  Demux9/1 -> Mux/6
  Demux8/1 -> Mux/5
  Demux1/2 -> MATLAB Function1/2(Yref)
  Demux/1 -> Mux/1
  Demux1/3 -> MATLAB Function3/2(Yref)
  MATLAB Function2/1(dX) -> Integrator1/1
  Demux3/1 -> MATLAB Function2/4(k)
  Demux2/4 -> MATLAB Function4/3(dYref)
  Demux4/1 -> Mux/7
  Demux2/2 -> MATLAB Function1/3(dYref)
  Mux/1 -> Out1/1
  In1/1 -> Derivative1/1, Demux1/1
  Mux1/1 -> Out2/1
  Selector/1 -> Demux/1
  Selector1/1 -> Demux5/1
  Selector2/1 -> Demux6/1
  Selector3/1 -> Demux7/1
  Selector4/1 -> Demux8/1
  Selector5/1 -> Demux9/1
  Selector6/1 -> Demux4/1
  Derivative1/1 -> Demux2/1
  Mux2/1 -> Out3/1
  MATLAB Function2/2(U) -> Mux2/1
  MATLAB Function1/2(U) -> Mux2/2
  MATLAB Function4/2(U) -> Mux2/4
  MATLAB Function3/2(U) -> Mux2/3
  MATLAB Function6/2(U) -> Mux2/6
  MATLAB Function5/2(U) -> Mux2/5
  MATLAB Function7/2(U) -> Mux2/7

== matlab function Ensamblaje2/Subsystem/MATLAB Function2 ==
  data: X input; dX output; Yref input; dYref input; k input; U output
function [dX,U]= motor_pid(X, Yref, dYref, k)
x1 = 0; x2 = 0;
%MATRICES DEL MOTOR
Ra = 11.24;
La = 2.713e-3;
Kb = 14.87e-3;
Kt = Kb;
bm = 2.01e-6;
Jm = 2779.56e-9;

A = [-Ra/La -Kb/La;Kt/Jm -bm/Jm];
B = [1/La;0];
C = [0 1];

E = Yref - C*X(2:3);
dE = dYref - C*A*X(2:3);

U = k(1)*E + k(2)*X(1) + k(3)*dE;

if(U > 48)
    U = 48;
    
elseif(U < -48)
    U = -48;
end

dX = [E; A*X(2:3) + B*U];

== matlab function Ensamblaje2/MATLAB Function ==
  data: x input; dX output; yref input; dYref input; t input
function dX = simulink_jacobiano(x, yref,dYref,t)

Ke = -5;

%Parametros del sistema
d = [0.2703 0 0.3644 0 0.3743 0 0.2295]; %metros
a = [0.069 0 0.069 0 0.01 0 0]; %metros
alpha = [-pi/2 pi/2 -pi/2 pi/2 -pi/2 pi/2 0]; %radianes

T = D_H(x(1:7),a,alpha,d,0,7);
J = jacobiano(T);
Jv = J(4:6,:);

e = yref - T{1,7}(1:3,4);
U = pinv(Jv)*(dYref - Ke*e);
%ODE's
dX = [U;Jv*U];

== matlab function Ensamblaje2/Subsystem/MATLAB Function1 ==
  data: X input; dX output; Yref input; dYref input; k input; U output
function [dX,U] = motor_pid(X, Yref, dYref, k)
x1 = 0; x2 = 0;
%MATRICES DEL MOTOR
Ra = 11.24;
La = 2.713e-3;
Kb = 14.87e-3;
Kt = Kb;
bm = 2.01e-6;
Jm = 2779.56e-9;

A = [-Ra/La -Kb/La;Kt/Jm -bm/Jm];
B = [1/La;0];
C = [0 1];

E = Yref - C*X(2:3);
dE = dYref - C*A*X(2:3);

U = k(1)*E + k(2)*X(1) + k(3)*dE;

if(U > 48)
    U = 48;
end

dX = [E; A*X(2:3) + B*U];

== matlab function Ensamblaje2/Subsystem/MATLAB Function3 ==
  data: X input; dX output; Yref input; dYref input; k input; U output
function [dX,U] = motor_pid(X, Yref, dYref, k)
x1 = 0; x2 = 0;
%MATRICES DEL MOTOR
Ra = 11.24;
La = 2.713e-3;
Kb = 14.87e-3;
Kt = Kb;
bm = 2.01e-6;
Jm = 2779.56e-9;

A = [-Ra/La -Kb/La;Kt/Jm -bm/Jm];
B = [1/La;0];
C = [0 1];

E = Yref - C*X(2:3);
dE = dYref - C*A*X(2:3);

U = k(1)*E + k(2)*X(1) + k(3)*dE;

if(U > 48)
    U = 48;
elseif(U < -48)
    U = -48;
end

dX = [E; A*X(2:3) + B*U];

== matlab function Ensamblaje2/Subsystem/MATLAB Function4 ==
  data: X input; dX output; Yref input; dYref input; k input; U output
function [dX,U] = motor_pid(X, Yref, dYref, k)
x1 = 0; x2 = 0;
%MATRICES DEL MOTOR
Ra = 11.24;
La = 2.713e-3;
Kb = 14.87e-3;
Kt = Kb;
bm = 2.01e-6;
Jm = 2779.56e-9;

A = [-Ra/La -Kb/La;Kt/Jm -bm/Jm];
B = [1/La;0];
C = [0 1];

E = Yref - C*X(2:3);
dE = dYref - C*A*X(2:3);

U = k(1)*E + k(2)*X(1) + k(3)*dE;

if(U > 48)
    U = 48;
    
elseif(U < -48)
    U = -48;
end

dX = [E; A*X(2:3) + B*U];

== matlab function Ensamblaje2/Subsystem/MATLAB Function5 ==
  data: X input; dX output; Yref input; dYref input; k input; U output
function [dX,U] = motor_pid(X, Yref, dYref, k)
x1 = 0; x2 = 0;
%MATRICES DEL MOTOR
Ra = 11.24;
La = 2.713e-3;
Kb = 14.87e-3;
Kt = Kb;
bm = 2.01e-6;
Jm = 2779.56e-9;

A = [-Ra/La -Kb/La;Kt/Jm -bm/Jm];
B = [1/La;0];
C = [0 1];

E = Yref - C*X(2:3);
dE = dYref - C*A*X(2:3);

U = k(1)*E + k(2)*X(1) + k(3)*dE;

if(U > 48)
    U = 48;
    
elseif(U < -48)
    U = -48;
end

dX = [E; A*X(2:3) + B*U];

== matlab function Ensamblaje2/Subsystem/MATLAB Function6 ==
  data: X input; dX output; Yref input; dYref input; k input; U output
function [dX,U] = motor_pid(X, Yref, dYref, k)
x1 = 0; x2 = 0;
%MATRICES DEL MOTOR
Ra = 11.24;
La = 2.713e-3;
Kb = 14.87e-3;
Kt = Kb;
bm = 2.01e-6;
Jm = 2779.56e-9;

A = [-Ra/La -Kb/La;Kt/Jm -bm/Jm];
B = [1/La;0];
C = [0 1];

E = Yref - C*X(2:3);
dE = dYref - C*A*X(2:3);

U = k(1)*E + k(2)*X(1) + k(3)*dE;

if(U > 48)
    U = 48;
    
elseif(U < -48)
    U = -48;
end

dX = [E; A*X(2:3) + B*U];

== matlab function Ensamblaje2/Subsystem/MATLAB Function7 ==
  data: X input; dX output; Yref input; dYref input; k input; U output
function [dX,U] = motor_pid(X, Yref, dYref, k)
x1 = 0; x2 = 0;
%MATRICES DEL MOTOR
Ra = 11.24;
La = 2.713e-3;
Kb = 14.87e-3;
Kt = Kb;
bm = 2.01e-6;
Jm = 2779.56e-9;

A = [-Ra/La -Kb/La;Kt/Jm -bm/Jm];
B = [1/La;0];
C = [0 1];

E = Yref - C*X(2:3);
dE = dYref - C*A*X(2:3);

U = k(1)*E + k(2)*X(1) + k(3)*dE;

if(U > 48)
    U = 48;
    
elseif(U < -48)
    U = -48;
end

dX = [E; A*X(2:3) + B*U];
